simulink library "SimplexPS_2015a_old"  (R2015a)
settings: Solver=ode45  SolverMode=SingleTasking  StartTime=0.0  StopTime=10.0  RelTol=1e-3
undefined symbols (not defined in the file): ang_r, Cf, DiscIntNeverNeededParam, initial, Lc, Lf, m, P_dc, Sbase, t0, Tm_pu, Ts, Vbase, w_droop, w_i, w_pll, w_tau, w_v, Wbase, wc, wfil, x0, Ybase, Zbase
libraries: powerlib x239, SimplexPS_ x81, SimplexPS_2015a x4
(part 5 of 5)

== system SimplexPS_2015a_old/SynchronousMachineFull_SMAVRPSSGOV (dq-Frame System Object)/PQ Calculation (dq-Frame) ==
  note: Power calculation.
      |
      | Author(s): Yitong Li
      |
      | Notes:
      |
      | The calculation is done in dq frame.
  vdq : Inport
  idq : Inport  Port=2
  Mux : Mux  Inputs=2
  Mux1 : Mux  Inputs=2
  P = vd*id+vq*iq : Fcn  Expr=u[1]*u[3]+u[2]*u[4]
  Q = -vd*iq+vq*id : Fcn  Expr=-u[1]*u[4]+u[2]*u[3]
  pq : Outport
  wires:
  Mux/1 -> pq/1
  P = vd*id+vq*iq/1 -> Mux/1
  vdq/1 -> Mux1/1
  idq/1 -> Mux1/2
  Mux1/1 -> P = vd*id+vq*iq/1, Q = -vd*iq+vq*id/1
  Q = -vd*iq+vq*id/1 -> Mux/2

== system SimplexPS_2015a_old/SynchronousMachineFull_SMAVRPSSGOV_FS (dq-Frame System Object)/PQ Calculation (dq-Frame) ==
  note: Power calculation.
      |
      | Author(s): Yitong Li
      |
      | Notes:
      |
      | The calculation is done in dq frame.
  vdq : Inport
  idq : Inport  Port=2
  Mux : Mux  Inputs=2
  Mux1 : Mux  Inputs=2
  P = vd*id+vq*iq : Fcn  Expr=u[1]*u[3]+u[2]*u[4]
  Q = -vd*iq+vq*id : Fcn  Expr=-u[1]*u[4]+u[2]*u[3]
  pq : Outport
  wires:
  Mux/1 -> pq/1
  P = vd*id+vq*iq/1 -> Mux/1
  vdq/1 -> Mux1/1
  idq/1 -> Mux1/2
  Mux1/1 -> P = vd*id+vq*iq/1, Q = -vd*iq+vq*id/1
  Q = -vd*iq+vq*id/1 -> Mux/2

== system SimplexPS_2015a_old/SynchronousMachineFull_SMGOV_FS (dq-Frame System Object)/PQ Calculation (dq-Frame) ==
  note: Power calculation.
      |
      | Author(s): Yitong Li
      |
      | Notes:
      |
      | The calculation is done in dq frame.
  vdq : Inport
  idq : Inport  Port=2
  Mux : Mux  Inputs=2
  Mux1 : Mux  Inputs=2
  P = vd*id+vq*iq : Fcn  Expr=u[1]*u[3]+u[2]*u[4]
  Q = -vd*iq+vq*id : Fcn  Expr=-u[1]*u[4]+u[2]*u[3]
  pq : Outport
  wires:
  Mux/1 -> pq/1
  P = vd*id+vq*iq/1 -> Mux/1
  vdq/1 -> Mux1/1
  idq/1 -> Mux1/2
  Mux1/1 -> P = vd*id+vq*iq/1, Q = -vd*iq+vq*id/1
  Q = -vd*iq+vq*id/1 -> Mux/2

== system SimplexPS_2015a_old/SynchronousMachineFull_SM_GOV (dq-Frame System Object)/PQ Calculation (dq-Frame) ==
  note: Power calculation.
      |
      | Author(s): Yitong Li
      |
      | Notes:
      |
      | The calculation is done in dq frame.
  vdq : Inport
  idq : Inport  Port=2
  Mux : Mux  Inputs=2
  Mux1 : Mux  Inputs=2
  P = vd*id+vq*iq : Fcn  Expr=u[1]*u[3]+u[2]*u[4]
  Q = -vd*iq+vq*id : Fcn  Expr=-u[1]*u[4]+u[2]*u[3]
  pq : Outport
  wires:
  Mux/1 -> pq/1
  P = vd*id+vq*iq/1 -> Mux/1
  vdq/1 -> Mux1/1
  idq/1 -> Mux1/2
  Mux1/1 -> P = vd*id+vq*iq/1, Q = -vd*iq+vq*id/1
  Q = -vd*iq+vq*id/1 -> Mux/2

== system SimplexPS_2015a_old/Three-Phase Signal/dq -> abc (Power-Invariant) ==
  dq : Inport
  theta : Inport  Port=2
  ->a : Fcn  Expr=cos(u(3))*u(1) - sin(u(3))*u(2)
  ->b : Fcn  Expr=cos(u(3)-2/3*pi)*u(1) - sin(u(3)-2/3*pi)*u(2)
  ->c : Fcn  Expr=cos(u(3)-4/3*pi)*u(1) - sin(u(3)-4/3*pi)*u(2)
  Gain : Gain  Gain=sqrt(2/3)
  Mux5 : Mux  Inputs=2
  Mux6 : Mux  Inputs=3
  abc : Outport
  wires:
  ->b/1 -> Mux6/2
  ->a/1 -> Mux6/1
  Gain/1 -> Mux5/1
  dq/1 -> Gain/1
  ->c/1 -> Mux6/3
  Mux6/1 -> abc/1
  Mux5/1 -> ->b/1, ->a/1, ->c/1
  theta/1 -> Mux5/2

== system SimplexPS_2015a_old/Grid-Following Inverter (Simulink Block)/Current Controller/PI-DT-Estimated d ==
  enable : Inport
  reference : Inport  Port=2
  initial : Inport  Port=3
  actual : Inport  Port=4
  Discrete-Time Integrator : DiscreteIntegrator  gainval=1  ExternalReset=rising  InitialConditionSource=external  InitialCondition=initial  SampleTime=Ts  LimitOutput=on  UpperSaturationLimit=xmax  LowerSaturationLimit=xmin  ICPrevOutput=DiscIntNeverNeededParam  ICPrevScaledInput=DiscIntNeverNeededParam
  Ierror : Sum  Inputs=+-
  Ki : Gain  Gain=Ki  SaturateOnIntegerOverflow=on  OutDataTypeStr=Inherit: Same as input  ParamDataTypeStr=Inherit: Same as input
  Kp : Gain  Gain=Kp  SaturateOnIntegerOverflow=on  OutDataTypeStr=Inherit: Same as input  ParamDataTypeStr=Inherit: Same as input
  Perror : Sum  Inputs=-+
  Product : Product  RndMeth=Zero
  Product1 : Product  RndMeth=Zero
  Saturation : Saturate  UpperLimit=xmax  LowerLimit=xmin
  Sum1 : Sum  SaturateOnIntegerOverflow=on
  Out : Outport
  wires:
  Saturation/1 -> Out/1
  Sum1/1 -> Saturation/1
  Ki/1 -> Discrete-Time Integrator/1
  Kp/1 -> Sum1/1
  Discrete-Time Integrator/1 -> Sum1/2
  enable/1 -> Discrete-Time Integrator/2, Product/2, Product1/2
  initial/1 -> Discrete-Time Integrator/3
  actual/1 -> Perror/1, Ierror/2
  reference/1 -> Perror/2, Ierror/1
  Perror/1 -> Product/1
  Product/1 -> Kp/1
  Ierror/1 -> Product1/1
  Product1/1 -> Ki/1

== system SimplexPS_2015a_old/Grid-Following Inverter (Simulink Block)/Current Controller/PI-DT-Estimated q ==
  actual : Inport
  initial : Inport  Port=2
  reference : Inport  Port=3
  enable : Inport  Port=4
  Discrete-Time Integrator : DiscreteIntegrator  gainval=1  ExternalReset=rising  InitialConditionSource=external  InitialCondition=initial  SampleTime=Ts  LimitOutput=on  UpperSaturationLimit=xmax  LowerSaturationLimit=xmin  ICPrevOutput=DiscIntNeverNeededParam  ICPrevScaledInput=DiscIntNeverNeededParam
  Ierror : Sum  Inputs=+-
  Ki : Gain  Gain=Ki  SaturateOnIntegerOverflow=on  OutDataTypeStr=Inherit: Same as input  ParamDataTypeStr=Inherit: Same as input
  Kp : Gain  Gain=Kp  SaturateOnIntegerOverflow=on  OutDataTypeStr=Inherit: Same as input  ParamDataTypeStr=Inherit: Same as input
  Perror : Sum  Inputs=-+
  Product : Product  RndMeth=Zero
  Product1 : Product  RndMeth=Zero
  Saturation : Saturate  UpperLimit=xmax  LowerLimit=xmin
  Sum1 : Sum  SaturateOnIntegerOverflow=on
  Out : Outport
  wires:
  Saturation/1 -> Out/1
  Sum1/1 -> Saturation/1
  Ki/1 -> Discrete-Time Integrator/1
  Kp/1 -> Sum1/1
  Discrete-Time Integrator/1 -> Sum1/2
  enable/1 -> Discrete-Time Integrator/2, Product/2, Product1/2
  initial/1 -> Discrete-Time Integrator/3
  actual/1 -> Ierror/2, Perror/1
  reference/1 -> Perror/2, Ierror/1
  Perror/1 -> Product/1
  Product/1 -> Kp/1
  Ierror/1 -> Product1/1
  Product1/1 -> Ki/1

== system SimplexPS_2015a_old/Grid-Forming Inverter (Simulink Block)/Current Controller/PI-DT-Estimated d ==
  enable : Inport
  reference : Inport  Port=2
  initial : Inport  Port=3
  actual : Inport  Port=4
  Discrete-Time Integrator : DiscreteIntegrator  gainval=1  ExternalReset=rising  InitialConditionSource=external  InitialCondition=initial  SampleTime=Ts  LimitOutput=on  UpperSaturationLimit=xmax  LowerSaturationLimit=xmin  ICPrevOutput=DiscIntNeverNeededParam  ICPrevScaledInput=DiscIntNeverNeededParam
  Ierror : Sum  Inputs=+-
  Ki : Gain  Gain=Ki  SaturateOnIntegerOverflow=on  OutDataTypeStr=Inherit: Same as input  ParamDataTypeStr=Inherit: Same as input
  Kp : Gain  Gain=Kp  SaturateOnIntegerOverflow=on  OutDataTypeStr=Inherit: Same as input  ParamDataTypeStr=Inherit: Same as input
  Perror : Sum  Inputs=-+
  Product : Product  RndMeth=Zero
  Product1 : Product  RndMeth=Zero
  Saturation : Saturate  UpperLimit=xmax  LowerLimit=xmin
  Sum1 : Sum  SaturateOnIntegerOverflow=on
  Out : Outport
  wires:
  Saturation/1 -> Out/1
  Sum1/1 -> Saturation/1
  Ki/1 -> Discrete-Time Integrator/1
  Kp/1 -> Sum1/1
  Discrete-Time Integrator/1 -> Sum1/2
  enable/1 -> Discrete-Time Integrator/2, Product/2, Product1/2
  initial/1 -> Discrete-Time Integrator/3
  actual/1 -> Perror/1, Ierror/2
  reference/1 -> Perror/2, Ierror/1
  Perror/1 -> Product/1
  Product/1 -> Kp/1
  Ierror/1 -> Product1/1
  Product1/1 -> Ki/1

== system SimplexPS_2015a_old/Grid-Forming Inverter (Simulink Block)/Current Controller/PI-DT-Estimated q ==
  actual : Inport
  initial : Inport  Port=2
  reference : Inport  Port=3
  enable : Inport  Port=4
  Discrete-Time Integrator : DiscreteIntegrator  gainval=1  ExternalReset=rising  InitialConditionSource=external  InitialCondition=initial  SampleTime=Ts  LimitOutput=on  UpperSaturationLimit=xmax  LowerSaturationLimit=xmin  ICPrevOutput=DiscIntNeverNeededParam  ICPrevScaledInput=DiscIntNeverNeededParam
  Ierror : Sum  Inputs=+-
  Ki : Gain  Gain=Ki  SaturateOnIntegerOverflow=on  OutDataTypeStr=Inherit: Same as input  ParamDataTypeStr=Inherit: Same as input
  Kp : Gain  Gain=Kp  SaturateOnIntegerOverflow=on  OutDataTypeStr=Inherit: Same as input  ParamDataTypeStr=Inherit: Same as input
  Perror : Sum  Inputs=-+
  Product : Product  RndMeth=Zero
  Product1 : Product  RndMeth=Zero
  Saturation : Saturate  UpperLimit=xmax  LowerLimit=xmin
  Sum1 : Sum  SaturateOnIntegerOverflow=on
  Out : Outport
  wires:
  Saturation/1 -> Out/1
  Sum1/1 -> Saturation/1
  Ki/1 -> Discrete-Time Integrator/1
  Kp/1 -> Sum1/1
  Discrete-Time Integrator/1 -> Sum1/2
  enable/1 -> Discrete-Time Integrator/2, Product/2, Product1/2
  initial/1 -> Discrete-Time Integrator/3
  actual/1 -> Ierror/2, Perror/1
  reference/1 -> Perror/2, Ierror/1
  Perror/1 -> Product/1
  Product/1 -> Kp/1
  Ierror/1 -> Product1/1
  Product1/1 -> Ki/1

== system SimplexPS_2015a_old/Grid-Forming Inverter (Simulink Block)/Voltage Controller/PI-DT-Estimated d ==
  enable : Inport
  reference : Inport  Port=2
  initial : Inport  Port=3
  actual : Inport  Port=4
  Discrete-Time Integrator : DiscreteIntegrator  gainval=1  ExternalReset=rising  InitialConditionSource=external  InitialCondition=initial  SampleTime=Ts  LimitOutput=on  UpperSaturationLimit=xmax  LowerSaturationLimit=xmin  ICPrevOutput=DiscIntNeverNeededParam  ICPrevScaledInput=DiscIntNeverNeededParam
  Ierror : Sum  Inputs=+-
  Ki : Gain  Gain=Ki  SaturateOnIntegerOverflow=on  OutDataTypeStr=Inherit: Same as input  ParamDataTypeStr=Inherit: Same as input
  Kp : Gain  Gain=Kp  SaturateOnIntegerOverflow=on  OutDataTypeStr=Inherit: Same as input  ParamDataTypeStr=Inherit: Same as input
  Perror : Sum  Inputs=-+
  Product : Product  RndMeth=Zero
  Product1 : Product  RndMeth=Zero
  Saturation : Saturate  UpperLimit=xmax  LowerLimit=xmin
  Sum1 : Sum  SaturateOnIntegerOverflow=on
  Out : Outport
  wires:
  Saturation/1 -> Out/1
  Sum1/1 -> Saturation/1
  Ki/1 -> Discrete-Time Integrator/1
  Kp/1 -> Sum1/1
  Discrete-Time Integrator/1 -> Sum1/2
  enable/1 -> Discrete-Time Integrator/2, Product/2, Product1/2
  initial/1 -> Discrete-Time Integrator/3
  actual/1 -> Perror/1, Ierror/2
  reference/1 -> Perror/2, Ierror/1
  Perror/1 -> Product/1
  Product/1 -> Kp/1
  Ierror/1 -> Product1/1
  Product1/1 -> Ki/1

== system SimplexPS_2015a_old/Grid-Forming Inverter (Simulink Block)/Voltage Controller/PI-DT-Estimated q ==
  actual : Inport
  initial : Inport  Port=2
  reference : Inport  Port=3
  enable : Inport  Port=4
  Discrete-Time Integrator : DiscreteIntegrator  gainval=1  ExternalReset=rising  InitialConditionSource=external  InitialCondition=initial  SampleTime=Ts  LimitOutput=on  UpperSaturationLimit=xmax  LowerSaturationLimit=xmin  ICPrevOutput=DiscIntNeverNeededParam  ICPrevScaledInput=DiscIntNeverNeededParam
  Ierror : Sum  Inputs=+-
  Ki : Gain  Gain=Ki  SaturateOnIntegerOverflow=on  OutDataTypeStr=Inherit: Same as input  ParamDataTypeStr=Inherit: Same as input
  Kp : Gain  Gain=Kp  SaturateOnIntegerOverflow=on  OutDataTypeStr=Inherit: Same as input  ParamDataTypeStr=Inherit: Same as input
  Perror : Sum  Inputs=-+
  Product : Product  RndMeth=Zero
  Product1 : Product  RndMeth=Zero
  Saturation : Saturate  UpperLimit=xmax  LowerLimit=xmin
  Sum1 : Sum  SaturateOnIntegerOverflow=on
  Out : Outport
  wires:
  Saturation/1 -> Out/1
  Sum1/1 -> Saturation/1
  Ki/1 -> Discrete-Time Integrator/1
  Kp/1 -> Sum1/1
  Discrete-Time Integrator/1 -> Sum1/2
  enable/1 -> Discrete-Time Integrator/2, Product/2, Product1/2
  initial/1 -> Discrete-Time Integrator/3
  actual/1 -> Ierror/2, Perror/1
  reference/1 -> Perror/2, Ierror/1
  Perror/1 -> Product/1
  Product/1 -> Kp/1
  Ierror/1 -> Product1/1
  Product1/1 -> Ki/1
